simulink model "Linearization"  (R2022a)
settings: Solver=VariableStepAuto  StartTime=0.0  StopTime=100  RelTol=1e-3
undefined symbols (not defined in the file): Aactuator, ac, AeroCoeff, ControlAllocation, DUmax, DUmin, EngineTable, F, fcs, ft, g, hground, IC, kg, LandingGear, Light, LPmethod, m, MIL, Mode_deflection_aileron, Mode_deflection_elevator, Mode_deflection_rudder, Mode_deflection_TVC_y, Mode_deflection_TVC_z, N, Ninv_2nozzle, Ninv_no_nozzle, PIController, s, Sensor, slug, state0, sysID_DAQ, sysID_OBES, Umax_2nozzle, Umax_no_nozzle, Umin_2nozzle, Umin_no_nozzle, WMM2020
libraries: aerolibconvert2 x19, slpidlib x6, simulink x6, sharedutil x4, aerolibatmos2 x3, aerolibwind2 x3, aerolibbdyn x3, aerolibgravity2 x2, sharedtransform x1
(part 1 of 9)
settings Model: Creator=user  LastModifiedBy=user
settings DataIOCC: ExternalInput=getinputstruct(op_trim1)  InitialState=getstatestruct(op_trim1)  LoadExternalInput=on  LoadInitialState=on  ReturnWorkspaceOutputs=off

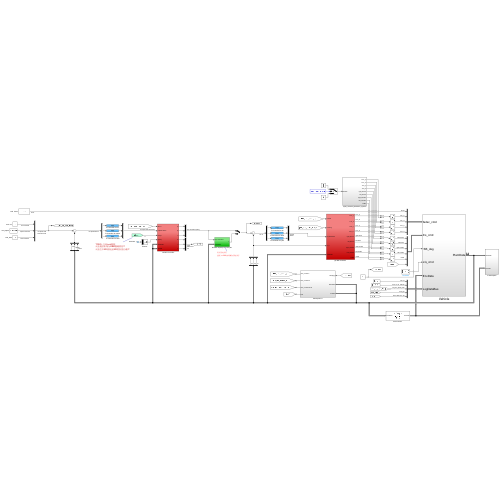
[thumbnail: Simulink's stored preview of the top-level diagram]
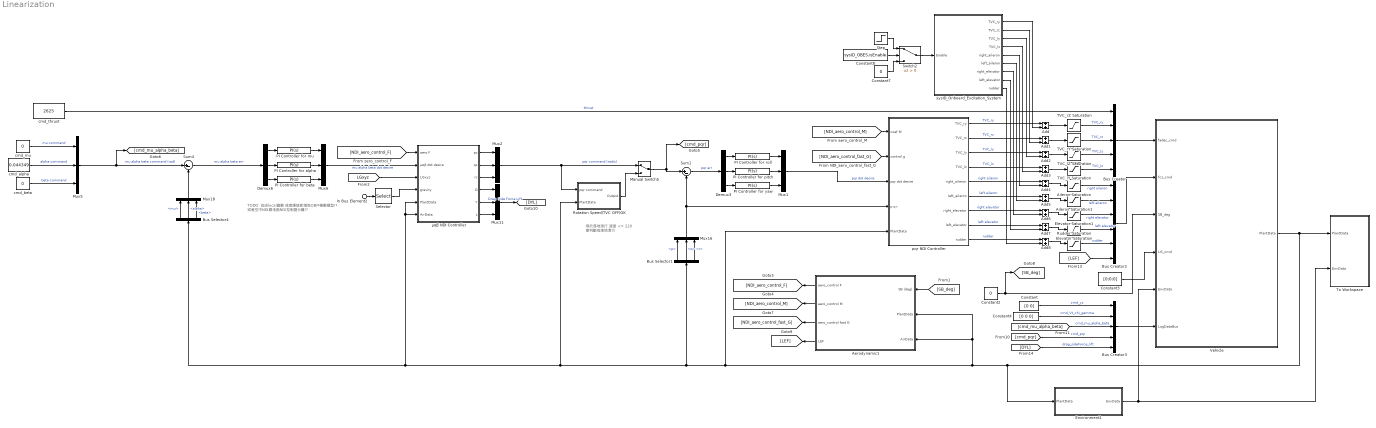
== system Linearization ==
  note: 用於落地滑行
      | 速度 <= 220 會判斷為落地滑行
  note: TODO: 改成local變數
      | 或者應該新增為OBM機載模型!?
      | 或者空中NDI跟地面NDI控制器分離!?
  In Bus Element2 : Inport  PortName=EnvData  Element=g
  Add{,1..8} (9 alike) : Sum
  Aerodynamic1 : Subsystem
  Aileron Saturation : Saturate  UpperLimit=Aactuator.aileron.AngleLimitUpper  LowerLimit=Aactuator.aileron.AngleLimitLower
  Aileron Saturation1 : Saturate  UpperLimit=Aactuator.aileron.AngleLimitUpper  LowerLimit=Aactuator.aileron.AngleLimitLower
  Bus Creator : BusCreator  Inputs=5
  Bus Creator2 : BusCreator  Inputs=6
  Bus Creator3 : BusCreator  Inputs=5
  Bus Selector1 : BusSelector  OutputSignals=p,q,r
  Bus Selector4 : BusSelector  OutputSignals=mu,alpha,beta
  Constant : Constant  Value=[0 0]
  Constant2 : Constant  Value=0
  Constant3 : Constant  Value=[0;0;0]
  Constant4 : Constant  Value=[0 0 0]
  Constant7 : Constant  Value=0
  Constant8 : Constant  Value=sysID_OBES.isEnable
  Demux3 : Demux  Outputs=3
  Demux6 : Demux  Outputs=3
  Elevator Saturation : Saturate  UpperLimit=Aactuator.elevator.AngleLimitUpper  LowerLimit=Aactuator.elevator.AngleLimitLower
  Elevator Saturation1 : Saturate  UpperLimit=Aactuator.elevator.AngleLimitUpper  LowerLimit=Aactuator.elevator.AngleLimitLower
  Environment1 : Subsystem
      mask Display:
      | image('aeroenvironment.bmp','center')
      | % 左側 "Icon transparency" 欄位已選擇 "Opaque with ports"，所以埠名稱會自動顯示，不用再宣告
      | % port_label('input',1,'PlantData')
      | % port_label('output',1,'EnvData')
  Manual Switch5 : ManualSwitch
  Mux{1..2,5..6,11,16,18} (7 alike) : Mux  Inputs=3
  PI Controller for alpha : slpidlib/PID Controller  Controller=PI  Form=Parallel  TimeDomain=Continuous-time  UseExternalTs=off  SampleTime=-1  IntegratorMethod=Forward Euler  FilterMethod=Forward Euler  ControllerParametersSource=internal  P=PIController.alpha.P  I=PIController.alpha.I  UseKiTs=off  D=0  N=100  UseFilter=on  TunerSelectOption=Transfer Function Based (PID Tuner App)  InitialConditionSource=internal  InitialConditionForIntegrator=0  InitialConditionForFilter=0  DifferentiatorICPrevScaledInput=0  ExternalReset=none  TrackingMode=off  Kt=1  LimitOutput=off  SatLimitsSource=internal  UpperSaturationLimit=inf  LowerSaturationLimit=-inf  LinearizeAsGain=on  AntiWindupMode=none  Kb=1  POutMin=[]  POutMax=[]  IOutMin=[]  IOutMax=[]  DOutMin=[]  DOutMax=[]  NOutMin=[]  NOutMax=[]  SumOutMin=[]  SumOutMax=[]  SaturationOutMin=[]  SaturationOutMax=[]  PParamMin=[]  PParamMax=[]  IParamMin=[]  IParamMax=[]  DParamMin=[]  DParamMax=[]  NParamMin=[]  NParamMax=[]  KbParamMin=[]  KbParamMax=[]  KtParamMin=[]  KtParamMax=[]  KbOutMin=[]  KbOutMax=[]  KtOutMin=[]  KtOutMax=[]  IntegratorOutMin=[]  IntegratorOutMax=[]  FilterOutMin=[]  FilterOutMax=[]  SumI1OutMin=[]  SumI1OutMax=[]  SumI2OutMin=[]  SumI2OutMax=[]  SumI3OutMin=[]  SumI3OutMax=[]  SumI4OutMin=[]  SumI4OutMax=[]  SumDOutMin=[]  SumDOutMax=[]  DifferentiatorOutMin=[]  DifferentiatorOutMax=[]  FilterDiffOutCoefMin=[]  FilterDiffOutCoefMax=[]  ReciprocalOutMin=[]  ReciprocalOutMax=[]  SumDenOutMin=[]  SumDenOutMax=[]  SumNumOutMin=[]  SumNumOutMax=[]  DivideOutMin=[]  DivideOutMax=[]  UdiffTsProdOutMin=[]  UdiffTsProdOutMax=[]  NTsProdOutMin=[]  NTsProdOutMax=[]  UintegralTsProdOutMin=[]  UintegralTsProdOutMax=[]  UngainTsProdOutMin=[]  UngainTsProdOutMax=[]  IntegratorContinuousStateAttributes=''  IntegratorStateMustResolveToSignalObject=off  IntegratorRTWStateStorageClass=Auto  FilterContinuousStateAttributes=''  FilterStateMustResolveToSignalObject=off  FilterRTWStateStorageClass=Auto  ParallelPVariant=InternalParameters  IdealPVariant=Disabled  IVariant=InternalParameters  DVariant=Disabled  IntegratorVariant=Continuous  SatVariant=Disabled  AWVariant=Passthrough  PCopyVariant=Disabled  TRVariant=Disabled  FdbkBlocksVariant=Forward  IdealPFdbkVariant=Disabled  SatFdbkVariant=Disabled  DerivativeFilterVariant=Disabled  NVariant=Disabled  NCopyVariant=Disabled_SignalSpec  FilterICVariant=Disabled  IntegratorICVariant=InternalICs  ExternalResetVariant=Disabled  TRSumVariant=Passthrough  SumFdbkVariant=Disabled  SumVariant=Sum_PI  TsampFilterVariant=InternalTs  TsampNgainVariant=Passthrough  TsampIntegralVariant=Passthrough  ExternalSaturationOutDataTypeStr=Inherit: Same as second input  aMode=0
  PI Controller for beta : slpidlib/PID Controller  Controller=PI  Form=Parallel  TimeDomain=Continuous-time  UseExternalTs=off  SampleTime=-1  IntegratorMethod=Forward Euler  FilterMethod=Forward Euler  ControllerParametersSource=internal  P=PIController.beta.P  I=PIController.beta.I  UseKiTs=off  D=0  N=100  UseFilter=on  TunerSelectOption=Transfer Function Based (PID Tuner App)  InitialConditionSource=internal  InitialConditionForIntegrator=0  InitialConditionForFilter=0  DifferentiatorICPrevScaledInput=0  ExternalReset=none  TrackingMode=off  Kt=1  LimitOutput=off  SatLimitsSource=internal  UpperSaturationLimit=inf  LowerSaturationLimit=-inf  LinearizeAsGain=on  AntiWindupMode=none  Kb=1  POutMin=[]  POutMax=[]  IOutMin=[]  IOutMax=[]  DOutMin=[]  DOutMax=[]  NOutMin=[]  NOutMax=[]  SumOutMin=[]  SumOutMax=[]  SaturationOutMin=[]  SaturationOutMax=[]  PParamMin=[]  PParamMax=[]  IParamMin=[]  IParamMax=[]  DParamMin=[]  DParamMax=[]  NParamMin=[]  NParamMax=[]  KbParamMin=[]  KbParamMax=[]  KtParamMin=[]  KtParamMax=[]  KbOutMin=[]  KbOutMax=[]  KtOutMin=[]  KtOutMax=[]  IntegratorOutMin=[]  IntegratorOutMax=[]  FilterOutMin=[]  FilterOutMax=[]  SumI1OutMin=[]  SumI1OutMax=[]  SumI2OutMin=[]  SumI2OutMax=[]  SumI3OutMin=[]  SumI3OutMax=[]  SumI4OutMin=[]  SumI4OutMax=[]  SumDOutMin=[]  SumDOutMax=[]  DifferentiatorOutMin=[]  DifferentiatorOutMax=[]  FilterDiffOutCoefMin=[]  FilterDiffOutCoefMax=[]  ReciprocalOutMin=[]  ReciprocalOutMax=[]  SumDenOutMin=[]  SumDenOutMax=[]  SumNumOutMin=[]  SumNumOutMax=[]  DivideOutMin=[]  DivideOutMax=[]  UdiffTsProdOutMin=[]  UdiffTsProdOutMax=[]  NTsProdOutMin=[]  NTsProdOutMax=[]  UintegralTsProdOutMin=[]  UintegralTsProdOutMax=[]  UngainTsProdOutMin=[]  UngainTsProdOutMax=[]  IntegratorContinuousStateAttributes=''  IntegratorStateMustResolveToSignalObject=off  IntegratorRTWStateStorageClass=Auto  FilterContinuousStateAttributes=''  FilterStateMustResolveToSignalObject=off  FilterRTWStateStorageClass=Auto  ParallelPVariant=InternalParameters  IdealPVariant=Disabled  IVariant=InternalParameters  DVariant=Disabled  IntegratorVariant=Continuous  SatVariant=Disabled  AWVariant=Passthrough  PCopyVariant=Disabled  TRVariant=Disabled  FdbkBlocksVariant=Forward  IdealPFdbkVariant=Disabled  SatFdbkVariant=Disabled  DerivativeFilterVariant=Disabled  NVariant=Disabled  NCopyVariant=Disabled_SignalSpec  FilterICVariant=Disabled  IntegratorICVariant=InternalICs  ExternalResetVariant=Disabled  TRSumVariant=Passthrough  SumFdbkVariant=Disabled  SumVariant=Sum_PI  TsampFilterVariant=InternalTs  TsampNgainVariant=Passthrough  TsampIntegralVariant=Passthrough  ExternalSaturationOutDataTypeStr=Inherit: Same as second input  aMode=0
  PI Controller for mu : slpidlib/PID Controller  Controller=PI  Form=Parallel  TimeDomain=Continuous-time  UseExternalTs=off  SampleTime=-1  IntegratorMethod=Forward Euler  FilterMethod=Forward Euler  ControllerParametersSource=internal  P=PIController.mu.P  I=PIController.mu.I  UseKiTs=off  D=0  N=100  UseFilter=on  TunerSelectOption=Transfer Function Based (PID Tuner App)  InitialConditionSource=internal  InitialConditionForIntegrator=0  InitialConditionForFilter=0  DifferentiatorICPrevScaledInput=0  ExternalReset=none  TrackingMode=off  Kt=1  LimitOutput=off  SatLimitsSource=internal  UpperSaturationLimit=inf  LowerSaturationLimit=-inf  LinearizeAsGain=on  AntiWindupMode=none  Kb=1  POutMin=[]  POutMax=[]  IOutMin=[]  IOutMax=[]  DOutMin=[]  DOutMax=[]  NOutMin=[]  NOutMax=[]  SumOutMin=[]  SumOutMax=[]  SaturationOutMin=[]  SaturationOutMax=[]  PParamMin=[]  PParamMax=[]  IParamMin=[]  IParamMax=[]  DParamMin=[]  DParamMax=[]  NParamMin=[]  NParamMax=[]  KbParamMin=[]  KbParamMax=[]  KtParamMin=[]  KtParamMax=[]  KbOutMin=[]  KbOutMax=[]  KtOutMin=[]  KtOutMax=[]  IntegratorOutMin=[]  IntegratorOutMax=[]  FilterOutMin=[]  FilterOutMax=[]  SumI1OutMin=[]  SumI1OutMax=[]  SumI2OutMin=[]  SumI2OutMax=[]  SumI3OutMin=[]  SumI3OutMax=[]  SumI4OutMin=[]  SumI4OutMax=[]  SumDOutMin=[]  SumDOutMax=[]  DifferentiatorOutMin=[]  DifferentiatorOutMax=[]  FilterDiffOutCoefMin=[]  FilterDiffOutCoefMax=[]  ReciprocalOutMin=[]  ReciprocalOutMax=[]  SumDenOutMin=[]  SumDenOutMax=[]  SumNumOutMin=[]  SumNumOutMax=[]  DivideOutMin=[]  DivideOutMax=[]  UdiffTsProdOutMin=[]  UdiffTsProdOutMax=[]  NTsProdOutMin=[]  NTsProdOutMax=[]  UintegralTsProdOutMin=[]  UintegralTsProdOutMax=[]  UngainTsProdOutMin=[]  UngainTsProdOutMax=[]  IntegratorContinuousStateAttributes=''  IntegratorStateMustResolveToSignalObject=off  IntegratorRTWStateStorageClass=Auto  FilterContinuousStateAttributes=''  FilterStateMustResolveToSignalObject=off  FilterRTWStateStorageClass=Auto  ParallelPVariant=InternalParameters  IdealPVariant=Disabled  IVariant=InternalParameters  DVariant=Disabled  IntegratorVariant=Continuous  SatVariant=Disabled  AWVariant=Passthrough  PCopyVariant=Disabled  TRVariant=Disabled  FdbkBlocksVariant=Forward  IdealPFdbkVariant=Disabled  SatFdbkVariant=Disabled  DerivativeFilterVariant=Disabled  NVariant=Disabled  NCopyVariant=Disabled_SignalSpec  FilterICVariant=Disabled  IntegratorICVariant=InternalICs  ExternalResetVariant=Disabled  TRSumVariant=Passthrough  SumFdbkVariant=Disabled  SumVariant=Sum_PI  TsampFilterVariant=InternalTs  TsampNgainVariant=Passthrough  TsampIntegralVariant=Passthrough  ExternalSaturationOutDataTypeStr=Inherit: Same as second input  aMode=0
  PI Controller for pitch : slpidlib/PID Controller  Controller=PI  Form=Parallel  TimeDomain=Continuous-time  UseExternalTs=off  SampleTime=-1  IntegratorMethod=Forward Euler  FilterMethod=Forward Euler  ControllerParametersSource=internal  P=PIController.q.P  I=PIController.q.I  UseKiTs=off  D=0  N=100  UseFilter=on  TunerSelectOption=Transfer Function Based (PID Tuner App)  InitialConditionSource=internal  InitialConditionForIntegrator=0  InitialConditionForFilter=0  DifferentiatorICPrevScaledInput=0  ExternalReset=none  TrackingMode=off  Kt=1  LimitOutput=off  SatLimitsSource=internal  UpperSaturationLimit=inf  LowerSaturationLimit=-inf  LinearizeAsGain=on  AntiWindupMode=none  Kb=1  POutMin=[]  POutMax=[]  IOutMin=[]  IOutMax=[]  DOutMin=[]  DOutMax=[]  NOutMin=[]  NOutMax=[]  SumOutMin=[]  SumOutMax=[]  SaturationOutMin=[]  SaturationOutMax=[]  PParamMin=[]  PParamMax=[]  IParamMin=[]  IParamMax=[]  DParamMin=[]  DParamMax=[]  NParamMin=[]  NParamMax=[]  KbParamMin=[]  KbParamMax=[]  KtParamMin=[]  KtParamMax=[]  KbOutMin=[]  KbOutMax=[]  KtOutMin=[]  KtOutMax=[]  IntegratorOutMin=[]  IntegratorOutMax=[]  FilterOutMin=[]  FilterOutMax=[]  SumI1OutMin=[]  SumI1OutMax=[]  SumI2OutMin=[]  SumI2OutMax=[]  SumI3OutMin=[]  SumI3OutMax=[]  SumI4OutMin=[]  SumI4OutMax=[]  SumDOutMin=[]  SumDOutMax=[]  DifferentiatorOutMin=[]  DifferentiatorOutMax=[]  FilterDiffOutCoefMin=[]  FilterDiffOutCoefMax=[]  ReciprocalOutMin=[]  ReciprocalOutMax=[]  SumDenOutMin=[]  SumDenOutMax=[]  SumNumOutMin=[]  SumNumOutMax=[]  DivideOutMin=[]  DivideOutMax=[]  UdiffTsProdOutMin=[]  UdiffTsProdOutMax=[]  NTsProdOutMin=[]  NTsProdOutMax=[]  UintegralTsProdOutMin=[]  UintegralTsProdOutMax=[]  UngainTsProdOutMin=[]  UngainTsProdOutMax=[]  IntegratorContinuousStateAttributes=''  IntegratorStateMustResolveToSignalObject=off  IntegratorRTWStateStorageClass=Auto  FilterContinuousStateAttributes=''  FilterStateMustResolveToSignalObject=off  FilterRTWStateStorageClass=Auto  ParallelPVariant=InternalParameters  IdealPVariant=Disabled  IVariant=InternalParameters  DVariant=Disabled  IntegratorVariant=Continuous  SatVariant=Disabled  AWVariant=Passthrough  PCopyVariant=Disabled  TRVariant=Disabled  FdbkBlocksVariant=Forward  IdealPFdbkVariant=Disabled  SatFdbkVariant=Disabled  DerivativeFilterVariant=Disabled  NVariant=Disabled  NCopyVariant=Disabled_SignalSpec  FilterICVariant=Disabled  IntegratorICVariant=InternalICs  ExternalResetVariant=Disabled  TRSumVariant=Passthrough  SumFdbkVariant=Disabled  SumVariant=Sum_PI  TsampFilterVariant=InternalTs  TsampNgainVariant=Passthrough  TsampIntegralVariant=Passthrough  ExternalSaturationOutDataTypeStr=Inherit: Same as second input  aMode=0
  PI Controller for roll : slpidlib/PID Controller  Controller=PI  Form=Parallel  TimeDomain=Continuous-time  UseExternalTs=off  SampleTime=-1  IntegratorMethod=Forward Euler  FilterMethod=Forward Euler  ControllerParametersSource=internal  P=PIController.p.P  I=PIController.p.I  UseKiTs=off  D=0  N=100  UseFilter=on  TunerSelectOption=Transfer Function Based (PID Tuner App)  InitialConditionSource=internal  InitialConditionForIntegrator=0  InitialConditionForFilter=0  DifferentiatorICPrevScaledInput=0  ExternalReset=none  TrackingMode=off  Kt=1  LimitOutput=off  SatLimitsSource=internal  UpperSaturationLimit=inf  LowerSaturationLimit=-inf  LinearizeAsGain=on  AntiWindupMode=none  Kb=1  POutMin=[]  POutMax=[]  IOutMin=[]  IOutMax=[]  DOutMin=[]  DOutMax=[]  NOutMin=[]  NOutMax=[]  SumOutMin=[]  SumOutMax=[]  SaturationOutMin=[]  SaturationOutMax=[]  PParamMin=[]  PParamMax=[]  IParamMin=[]  IParamMax=[]  DParamMin=[]  DParamMax=[]  NParamMin=[]  NParamMax=[]  KbParamMin=[]  KbParamMax=[]  KtParamMin=[]  KtParamMax=[]  KbOutMin=[]  KbOutMax=[]  KtOutMin=[]  KtOutMax=[]  IntegratorOutMin=[]  IntegratorOutMax=[]  FilterOutMin=[]  FilterOutMax=[]  SumI1OutMin=[]  SumI1OutMax=[]  SumI2OutMin=[]  SumI2OutMax=[]  SumI3OutMin=[]  SumI3OutMax=[]  SumI4OutMin=[]  SumI4OutMax=[]  SumDOutMin=[]  SumDOutMax=[]  DifferentiatorOutMin=[]  DifferentiatorOutMax=[]  FilterDiffOutCoefMin=[]  FilterDiffOutCoefMax=[]  ReciprocalOutMin=[]  ReciprocalOutMax=[]  SumDenOutMin=[]  SumDenOutMax=[]  SumNumOutMin=[]  SumNumOutMax=[]  DivideOutMin=[]  DivideOutMax=[]  UdiffTsProdOutMin=[]  UdiffTsProdOutMax=[]  NTsProdOutMin=[]  NTsProdOutMax=[]  UintegralTsProdOutMin=[]  UintegralTsProdOutMax=[]  UngainTsProdOutMin=[]  UngainTsProdOutMax=[]  IntegratorContinuousStateAttributes=''  IntegratorStateMustResolveToSignalObject=off  IntegratorRTWStateStorageClass=Auto  FilterContinuousStateAttributes=''  FilterStateMustResolveToSignalObject=off  FilterRTWStateStorageClass=Auto  ParallelPVariant=InternalParameters  IdealPVariant=Disabled  IVariant=InternalParameters  DVariant=Disabled  IntegratorVariant=Continuous  SatVariant=Disabled  AWVariant=Passthrough  PCopyVariant=Disabled  TRVariant=Disabled  FdbkBlocksVariant=Forward  IdealPFdbkVariant=Disabled  SatFdbkVariant=Disabled  DerivativeFilterVariant=Disabled  NVariant=Disabled  NCopyVariant=Disabled_SignalSpec  FilterICVariant=Disabled  IntegratorICVariant=InternalICs  ExternalResetVariant=Disabled  TRSumVariant=Passthrough  SumFdbkVariant=Disabled  SumVariant=Sum_PI  TsampFilterVariant=InternalTs  TsampNgainVariant=Passthrough  TsampIntegralVariant=Passthrough  ExternalSaturationOutDataTypeStr=Inherit: Same as second input  aMode=0
  PI Controller for yaw : slpidlib/PID Controller  Controller=PI  Form=Parallel  TimeDomain=Continuous-time  UseExternalTs=off  SampleTime=-1  IntegratorMethod=Forward Euler  FilterMethod=Forward Euler  ControllerParametersSource=internal  P=PIController.r.P  I=PIController.r.I  UseKiTs=off  D=0  N=100  UseFilter=on  TunerSelectOption=Transfer Function Based (PID Tuner App)  InitialConditionSource=internal  InitialConditionForIntegrator=0  InitialConditionForFilter=0  DifferentiatorICPrevScaledInput=0  ExternalReset=none  TrackingMode=off  Kt=1  LimitOutput=off  SatLimitsSource=internal  UpperSaturationLimit=inf  LowerSaturationLimit=-inf  LinearizeAsGain=on  AntiWindupMode=none  Kb=1  POutMin=[]  POutMax=[]  IOutMin=[]  IOutMax=[]  DOutMin=[]  DOutMax=[]  NOutMin=[]  NOutMax=[]  SumOutMin=[]  SumOutMax=[]  SaturationOutMin=[]  SaturationOutMax=[]  PParamMin=[]  PParamMax=[]  IParamMin=[]  IParamMax=[]  DParamMin=[]  DParamMax=[]  NParamMin=[]  NParamMax=[]  KbParamMin=[]  KbParamMax=[]  KtParamMin=[]  KtParamMax=[]  KbOutMin=[]  KbOutMax=[]  KtOutMin=[]  KtOutMax=[]  IntegratorOutMin=[]  IntegratorOutMax=[]  FilterOutMin=[]  FilterOutMax=[]  SumI1OutMin=[]  SumI1OutMax=[]  SumI2OutMin=[]  SumI2OutMax=[]  SumI3OutMin=[]  SumI3OutMax=[]  SumI4OutMin=[]  SumI4OutMax=[]  SumDOutMin=[]  SumDOutMax=[]  DifferentiatorOutMin=[]  DifferentiatorOutMax=[]  FilterDiffOutCoefMin=[]  FilterDiffOutCoefMax=[]  ReciprocalOutMin=[]  ReciprocalOutMax=[]  SumDenOutMin=[]  SumDenOutMax=[]  SumNumOutMin=[]  SumNumOutMax=[]  DivideOutMin=[]  DivideOutMax=[]  UdiffTsProdOutMin=[]  UdiffTsProdOutMax=[]  NTsProdOutMin=[]  NTsProdOutMax=[]  UintegralTsProdOutMin=[]  UintegralTsProdOutMax=[]  UngainTsProdOutMin=[]  UngainTsProdOutMax=[]  IntegratorContinuousStateAttributes=''  IntegratorStateMustResolveToSignalObject=off  IntegratorRTWStateStorageClass=Auto  FilterContinuousStateAttributes=''  FilterStateMustResolveToSignalObject=off  FilterRTWStateStorageClass=Auto  ParallelPVariant=InternalParameters  IdealPVariant=Disabled  IVariant=InternalParameters  DVariant=Disabled  IntegratorVariant=Continuous  SatVariant=Disabled  AWVariant=Passthrough  PCopyVariant=Disabled  TRVariant=Disabled  FdbkBlocksVariant=Forward  IdealPFdbkVariant=Disabled  SatFdbkVariant=Disabled  DerivativeFilterVariant=Disabled  NVariant=Disabled  NCopyVariant=Disabled_SignalSpec  FilterICVariant=Disabled  IntegratorICVariant=InternalICs  ExternalResetVariant=Disabled  TRSumVariant=Passthrough  SumFdbkVariant=Disabled  SumVariant=Sum_PI  TsampFilterVariant=InternalTs  TsampNgainVariant=Passthrough  TsampIntegralVariant=Passthrough  ExternalSaturationOutDataTypeStr=Inherit: Same as second input  aMode=0
  Rotation Speed(TVC OFF)OK : Subsystem
  Rudder Saturation : Saturate  UpperLimit=Aactuator.rudder.AngleLimitUpper  LowerLimit=Aactuator.rudder.AngleLimitLower
  Selector : Selector  InputPortWidth=3  IndexOptions=Index vector (dialog)  Indices=3  OutputSizes=1
  Step : Step  Time=sysID_OBES.start_time  SampleTime=0
  Sum1 : Sum  Inputs=|+-
  Sum4 : Sum  Inputs=|+-
  Switch2 : Switch  Criteria=u2 > Threshold  SaturateOnIntegerOverflow=off  InputSameDT=off
  TVC_lY Saturation : Saturate  UpperLimit=Aactuator.TVC_Z.AngleLimitUpper  LowerLimit=Aactuator.TVC_Z.AngleLimitLower
  TVC_lZ Saturation : Saturate  UpperLimit=Aactuator.TVC_Y.AngleLimitUpper  LowerLimit=Aactuator.TVC_Y.AngleLimitLower
  TVC_rY Saturation : Saturate  UpperLimit=Aactuator.TVC_Z.AngleLimitUpper  LowerLimit=Aactuator.TVC_Z.AngleLimitLower
  TVC_rZ Saturation : Saturate  UpperLimit=Aactuator.TVC_Y.AngleLimitUpper  LowerLimit=Aactuator.TVC_Y.AngleLimitLower
  To Workspace : Subsystem
  Vehicle : Subsystem
  cmd_alpha : Constant  Value=0.044349
  cmd_beta : Constant  Value=0
  cmd_mu : Constant  Value=0
  cmd_thrust : Constant  Value=2625
  pqr NDI Controller : Subsystem  VariantControl=TVC ON
  sysID_Onboard_Excitation_System : Subsystem
  μαβ NDI Controller : Subsystem
  wires:
  Rudder Saturation/1 -> Bus Creator2/5  "rudder"
  Vehicle/1(PlantData) -> Environment1/1(PlantData), μαβ NDI Controller/5(PlantData), μαβ NDI Controller/6(AirData), Bus Selector4/1, Rotation Speed(TVC OFF)OK/2(PlantData), Bus Selector1/1, pqr NDI Controller/5(PlantData), Aerodynamic1/2(PlantData), Aerodynamic1/3(AirData), To Workspace/1(PlantData)
  Add3/1 -> TVC_lY Saturation/1
  Constant8/1 -> Switch2/2
  μαβ NDI Controller/5(Y) -> Mux11/2
  [LEF] -> Bus Creator2/6
  Manual Switch5/1 -> [cmd_pqr], Sum1/1
  Mux1/1 -> pqr NDI Controller/3(pqr dot desire)  "pqr dot desire"
  Add1/1 -> TVC_rY Saturation/1
  pqr NDI Controller/3("TVC_ly ") -> Add2/1  "TVC_ly"
  Rotation Speed(TVC OFF)OK/1(Output) -> Manual Switch5/2
  μαβ NDI Controller/6(L) -> Mux11/3
  [NDI_aero_control_fast_G] -> pqr NDI Controller/2(control g)
  pqr NDI Controller/8(left_elevator) -> Add7/1  "left elevator"
  pqr NDI Controller/5(right_aileron) -> Add4/1  "right aileron"
  [NDI_aero_control_F] -> μαβ NDI Controller/1(aero F)
  [NDI_aero_control_M] -> pqr NDI Controller/1(coef M)
  pqr NDI Controller/2(TVC_rz) -> Add1/1  "TVC_rz"
  Bus Selector1/1 -> Mux16/1  "<p>"
  Step/1 -> Switch2/1
  Mux2/1 -> Manual Switch5/1, Rotation Speed(TVC OFF)OK/1(pqr command)  "pqr command (rad/s)"
  TVC_lY Saturation/1 -> Bus Creator/5  "TVC_lz"
  Add7/1 -> Elevator Saturation/1
  Add2/1 -> TVC_lZ Saturation/1
  Demux6/2 -> PI Controller for alpha/1
  pqr NDI Controller/7(right_elevator) -> Add6/1  "right elevator"
  pqr NDI Controller/6(left_aileron) -> Add5/1  "left aileron"
  Add5/1 -> Aileron Saturation1/1
  μαβ NDI Controller/3(rc) -> Mux2/3
  pqr NDI Controller/1("TVC_ry ") -> Add/1  "TVC_ry"
  Add/1 -> TVC_rZ Saturation/1
  sysID_Onboard_Excitation_System/4(TVC_lz) -> Add3/2
  TVC_rY Saturation/1 -> Bus Creator/3  "TVC_rz"
  sysID_Onboard_Excitation_System/2(TVC_rz) -> Add1/2
  Constant7/1 -> Switch2/3
  Switch2/1 -> sysID_Onboard_Excitation_System/1(Enable)
  Add4/1 -> Aileron Saturation/1
  sysID_Onboard_Excitation_System/9(rudder) -> Add8/2
  Aileron Saturation1/1 -> Bus Creator2/2  "left aileron"
  [LGxyz] -> μαβ NDI Controller/3(LGxyz)
  PI Controller for mu/1 -> Mux6/1
  TVC_lZ Saturation/1 -> Bus Creator/4  "TVC_ly"
  Elevator Saturation1/1 -> Bus Creator2/3  "right elevator"
  Bus Creator2/1 -> Vehicle/2(fcs_cmd)
  TVC_rZ Saturation/1 -> Bus Creator/2  "TVC_ry"
  Elevator Saturation/1 -> Bus Creator2/4  "left elevator"
  Bus Creator/1 -> Vehicle/1(fadec_cmd)
  sysID_Onboard_Excitation_System/8(left_elevator) -> Add7/2
  μαβ NDI Controller/4(D) -> Mux11/1
  μαβ NDI Controller/2(qc) -> Mux2/2
  sysID_Onboard_Excitation_System/1(TVC_ry) -> Add/2
  Add8/1 -> Rudder Saturation/1
  Bus Selector4/1 -> Mux18/1  "<mu>"
  Aerodynamic1/4(LEF) -> [LEF]
  PI Controller for alpha/1 -> Mux6/2
  Demux3/3 -> PI Controller for yaw/1
  sysID_Onboard_Excitation_System/7(right_elevator) -> Add6/2
  Demux6/1 -> PI Controller for mu/1
  Mux6/1 -> μαβ NDI Controller/2(μαβ dot desire)  "mu alpha beta dot desire"
  Bus Selector1/2 -> Mux16/2  "<q>"
  Bus Selector4/2 -> Mux18/2  "<alpha>"
  Add6/1 -> Elevator Saturation1/1
  Aerodynamic1/2(aero_control M) -> [NDI_aero_control_M]
  Mux18/1 -> Sum4/2
  Mux11/1 -> [DYL]  "Drag  Side Force Lift"
  Demux6/3 -> PI Controller for beta/1
  sysID_Onboard_Excitation_System/3(TVC_ly) -> Add2/2
  Demux3/1 -> PI Controller for roll/1
  [SB_deg] -> Aerodynamic1/1(SB (deg))
  Sum1/1 -> Demux3/1  "pqr err"
  PI Controller for beta/1 -> Mux6/3
  Mux16/1 -> pqr NDI Controller/4(p q r), Sum1/2
  sysID_Onboard_Excitation_System/5(right_aileron) -> Add4/2
  In Bus Element2/1 -> Selector/1
  Selector/1 -> μαβ NDI Controller/4(gravity)
  Bus Selector1/3 -> Mux16/3  "<r>"
  Bus Selector4/3 -> Mux18/3  "<beta>"
  Sum4/1 -> Demux6/1  "mu alpha beta err"
  pqr NDI Controller/4("TVC_lz ") -> Add3/1  "TVC_lz"
  Mux5/1 -> [cmd_mu_alpha_beta], Sum4/1  "mu alpha beta command (rad)"
  sysID_Onboard_Excitation_System/6(left_aileron) -> Add5/2
  PI Controller for pitch/1 -> Mux1/2
  PI Controller for yaw/1 -> Mux1/3
  Aerodynamic1/1(aero_control F) -> [NDI_aero_control_F]
  Aileron Saturation/1 -> Bus Creator2/1  "right aileron"
  PI Controller for roll/1 -> Mux1/1
  μαβ NDI Controller/1(pc) -> Mux2/1
  Demux3/2 -> PI Controller for pitch/1
  Aerodynamic1/3(aero_control fast G) -> [NDI_aero_control_fast_G]
  pqr NDI Controller/9(rudder) -> Add8/1  "rudder"
  Constant2/1 -> [SB_deg], Vehicle/3(" SB_deg")
  [cmd_mu_alpha_beta] -> Bus Creator3/3  "cmd_mu_alpha_beta"
  Bus Creator3/1 -> Vehicle/6(LogDataBus)
  Constant/1 -> Bus Creator3/1  "cmd_yz"
  Constant4/1 -> Bus Creator3/2  "cmd_Vt_chi_gamma"
  [cmd_pqr] -> Bus Creator3/4  "cmd_pqr"
  [DYL] -> Bus Creator3/5  "drag_sideForce_lift"
  Constant3/1 -> Vehicle/4(LG_cmd)
  cmd_beta/1 -> Mux5/3  "beta command"
  cmd_alpha/1 -> Mux5/2  "alpha command"
  cmd_mu/1 -> Mux5/1  "mu command"
  cmd_thrust/1 -> Bus Creator/1  "thrust"
  Environment1/1(EnvData) -> To Workspace/2(EnvData), Vehicle/5(EnvData)

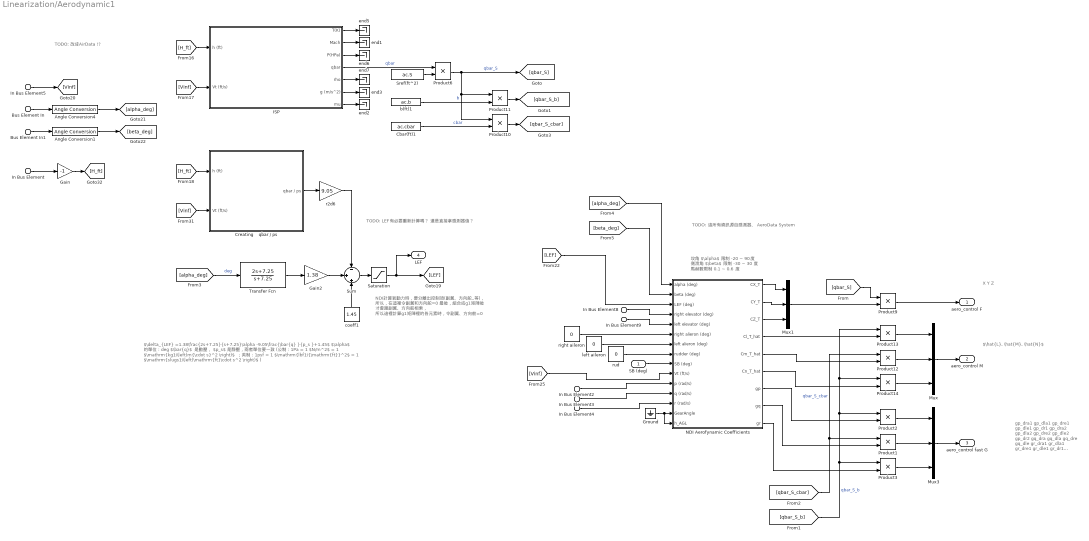
== system Linearization/Aerodynamic1 ==
  note: NDI計算氣動力時，要分離出控制項(副翼、方向舵..等)，
      | 所以，在這裡令副翼和方向舵=0
      | 最後，組合成g1矩陣後 才會跟副翼、方向舵相乘，
      | 所以這裡計算g1矩陣裡的各元素時，令副翼、方向舵=0
  note: TODO: LEF有必要重新計算嗎？
      | 還是直接拿感測器值？
  note: X
      | Y
      | Z
  note: $\delta_{LEF} =1.38\frac{2s+7.25}{s+7.25}\alpha -9.05\frac{\bar{q} }{p_s }+1.45$
      | $\alpha$ 的單位：deg
      | $\bar{q}$ 是動壓， $p_s$ 是靜壓，兩者單位要一致 (公制：1Pa = 1 $N/m^2$ = 1 $\mathrm{kg}/\left(m{\cdot s}^2 \right)$ ；英制：1psf = 1 $\mathrm{lbf}/{\mathrm{ft}}^2$ = 1 $\mathrm{slugs}/\left(\mathrm{ft}\cdot s^2 \right)$ )
  note: $\hat{L}, \hat{M}, \hat{N}$
  note: TODO: 這所有資訊源自感測器、
      | AeroData System
  note: TODO: 改成AirData !?
  note: 攻角 $\alpha$ 限制 -20 ~ 90度
      | 側滑角 $\beta$ 限制 -30 ~ 30 度
      | 馬赫數限制 0.1 ~ 0.6 度
  note: gp_dra1
      | gp_dla1
      | gp_dre1
      | gp_dle1
      | gp_dr1
      | gp_dra2
      | gp_dla2
      | gp_dre2
      | gp_dle2
      | gp_dr2
      |
      | gq_dra
      | gq_dla
      | gq_dre
      | gq_dle
      |
      | gr_dra1
      | gr_dla1
      | gr_dre1
      | gr_dle1
      | gr_dr1
      | gr_dra2
      | gr_dla2
      | gr_dre2
      | gr_dle2
      | gr_dr2
  SB (deg) : Inport  Unit=deg
  In Bus Element : Inport  Port=2  PortName=PlantData  Element=altitude
  In Bus Element8 : Inport  Port=2  PortName=PlantData  Element=AeroActBus.right Elevator_deg
  In Bus Element9 : Inport  Port=2  PortName=PlantData  Element=AeroActBus.left Elevator_deg
  In Bus Element2 : Inport  Port=2  PortName=PlantData  Element=p
  In Bus Element3 : Inport  Port=2  PortName=PlantData  Element=q
  In Bus Element4 : Inport  Port=2  PortName=PlantData  Element=r
  In Bus Element5 : Inport  Port=2  PortName=PlantData  Element=Vt
  Bus Element In : Inport  Port=3  PortName=AirData  Element=alpha
  Bus Element In1 : Inport  Port=3  PortName=AirData  Element=beta
  Angle Conversion1 : aerolibconvert2/Angle Conversion  IU=rad  OU=deg
  Angle Conversion4 : aerolibconvert2/Angle Conversion  IU=rad  OU=deg
  Cbar(ft)1 : Constant  Value=ac.cbar
  Creating    qbar / ps : Subsystem
  Gain : Gain  Gain=-1
  Gain2 : Gain  Gain=1.38  SaturateOnIntegerOverflow=on  OutDataTypeStr=Inherit: Same as input  ParamDataTypeStr=Inherit: Same as input
  Ground : Ground
  "ISP " : Subsystem
  Mux : Mux  Inputs=3
  Mux1 : Mux  Inputs=3
  Mux3 : Mux  Inputs=3
  NDI Aerofynamic Coefficients : Subsystem
  Product{1..3,6,9..14} (10 alike) : Product
  Saturation : Saturate  UpperLimit=Aactuator.LEF.AngleLimitUpper  LowerLimit=Aactuator.LEF.AngleLimitLower
  Sref(ft^2) : Constant  Value=ac.S
  Sum : Sum  Inputs=-|+|+  InputSameDT=on  SaturateOnIntegerOverflow=on  OutDataTypeStr=Inherit: Same as first input
  Transfer Fcn : TransferFcn  Numerator=[2 7.25]  Denominator=[1 7.25]
  b(ft)1 : Constant  Value=ac.b
  coeff1 : Constant  Value=1.45
  end{1..3,5..7} (6 alike) : Terminator
  left aileron : Constant  Value=0
  r2d6 : Gain  Gain=9.05  SaturateOnIntegerOverflow=on  OutDataTypeStr=Inherit: Same as input  ParamDataTypeStr=Inherit: Same as input
  right aileron : Constant  Value=0
  rud : Constant  Value=0
  aero_control F : Outport  VectorParamsAs1DForOutWhenUnconnected=off
  aero_control M : Outport  Port=2  VectorParamsAs1DForOutWhenUnconnected=off
  aero_control fast G : Outport  Port=3  VectorParamsAs1DForOutWhenUnconnected=off
  LEF : Outport  Port=4
  wires:
  [Vinf] -> "ISP "/2(Vt (ft/s))
  "ISP "/2("Mach ") -> end1/1
  "ISP "/7(mu) -> end2/1
  "ISP "/6(g (m/s^2)) -> end3/1
  "ISP "/5(rho) -> end7/1
  "ISP "/4("qbar ") -> Product6/1  "qbar"
  "ISP "/3(P(HPa)) -> end6/1
  "ISP "/1(T(K)) -> end5/1
  r2d6/1 -> Sum/1
  Creating    qbar / ps/1(qbar / ps) -> r2d6/1
  [alpha_deg] -> Transfer Fcn/1  "deg"
  [Vinf] -> Creating    qbar / ps/2(Vt (ft/s))
  coeff1/1 -> Sum/3
  [H_ft] -> Creating    qbar / ps/1(h (ft))
  [H_ft] -> "ISP "/1(h (ft))
  Sum/1 -> Saturation/1
  Saturation/1 -> LEF/1, [LEF]
  Transfer Fcn/1 -> Gain2/1
  In Bus Element/1 -> Gain/1
  Gain/1 -> [H_ft]
  Cbar(ft)1/1 -> Product10/2  "cbar"
  b(ft)1/1 -> Product11/2  "b"
  Sref(ft^2)/1 -> Product6/2
  Product10/1 -> [qbar_S_cbar]
  Product6/1 -> Product11/1, Product10/1, [qbar_S]  "qbar_S"
  Product11/1 -> [qbar_S_b]
  [qbar_S] -> Product9/1
  Product9/1 -> aero_control F/1
  Product12/1 -> Mux/2
  Product13/1 -> Mux/1
  Product14/1 -> Mux/3
  Mux/1 -> aero_control M/1
  NDI Aerofynamic Coefficients/4(Cl_T_hat) -> Product13/2
  NDI Aerofynamic Coefficients/5(Cm_T_hat) -> Product12/2
  NDI Aerofynamic Coefficients/6(Cn_T_hat) -> Product14/2
  NDI Aerofynamic Coefficients/1(CX_T) -> Mux1/1
  NDI Aerofynamic Coefficients/2(CY_T) -> Mux1/2
  NDI Aerofynamic Coefficients/3(CZ_T) -> Mux1/3
  Mux1/1 -> Product9/2
  [qbar_S_b] -> Product13/1, Product14/1, Product2/1, Product3/1  "qbar_S_b"
  Product3/1 -> Mux3/3
  Product1/1 -> Mux3/2
  Product2/1 -> Mux3/1
  NDI Aerofynamic Coefficients/7(gp) -> Product2/2
  [qbar_S_cbar] -> Product12/1, Product1/1  "qbar_S_cbar"
  NDI Aerofynamic Coefficients/9(gr) -> Product3/2
  NDI Aerofynamic Coefficients/8(gq) -> Product1/2
  Mux3/1 -> aero_control fast G/1
  [Vinf] -> NDI Aerofynamic Coefficients/10(Vt (ft/s))
  SB (deg)/1 -> NDI Aerofynamic Coefficients/9(SB (deg))
  [LEF] -> NDI Aerofynamic Coefficients/3(LEF (deg))
  [beta_deg] -> NDI Aerofynamic Coefficients/2(beta (deg))
  [alpha_deg] -> NDI Aerofynamic Coefficients/1(alpha (deg))
  In Bus Element2/1 -> NDI Aerofynamic Coefficients/11(p (rad/s))
  In Bus Element3/1 -> NDI Aerofynamic Coefficients/12(q (rad/s))
  In Bus Element4/1 -> NDI Aerofynamic Coefficients/13(r (rad/s))
  Ground/1 -> NDI Aerofynamic Coefficients/14(GearAngle), NDI Aerofynamic Coefficients/15(h_AGL)
  Gain2/1 -> Sum/2
  Bus Element In/1 -> Angle Conversion4/1
  Angle Conversion4/1 -> [alpha_deg]
  Angle Conversion1/1 -> [beta_deg]
  Bus Element In1/1 -> Angle Conversion1/1
  In Bus Element5/1 -> [Vinf]
  In Bus Element8/1 -> NDI Aerofynamic Coefficients/4(right elevator (deg))
  In Bus Element9/1 -> NDI Aerofynamic Coefficients/5(left elevator (deg))
  right aileron/1 -> NDI Aerofynamic Coefficients/6(right alieron (deg))
  left aileron/1 -> NDI Aerofynamic Coefficients/7(left alieron (deg))
  rud/1 -> NDI Aerofynamic Coefficients/8(rudder (deg))

== system Linearization/Environment1 ==
  note: p, q, r
  note: u, v, w
  note: Wind Models
  note: Atmosphere Model
  note: Altitude must be less than 20000 m (approximately 65620 feet).
  note: 建模注意： EnvData Bus 內要指定公制/英制單位
  note: Magnetic Field
  note: Gravity Model
  note: TODO: 改用這個現成模塊...
      | 但NDI控制器內的重力g是用常數，將產生誤差...
  note: TODO: 改用這個現成模塊...
      | 參考MATLAB Help範例 Quadcopter Project
  note: TODO: 改用現成模塊，改成英制。
      | NDI控制器，不會產生誤差，因為可轉成C程式碼
  note: TODO: 參考MATLAB Help範例 HL-20
      | 將風速效應加到氣動力攻角、側滑角、qbar、Mach、V
  In Bus Element3 : Inport  PortName=PlantData  Element=Vt
  In Bus Element4 : Inport  PortName=PlantData  Element=Vt
  In Bus Element5 : Inport  PortName=PlantData  Element=Vt
  In Bus Element : Inport  PortName=PlantData  Element=DCM_be
  In Bus Element1 : Inport  PortName=PlantData  Element=altitude
  In Bus Element2 : Inport  PortName=PlantData  Element=altitude
  COESA Atmosphere Model : aerolibatmos2/COESA Atmosphere Model  Commented=on  units=English (Velocity in ft/s)  spec=1976 COESA-extended U.S. Standard Atmosphere  model=Profile  profile_var=High temperature  profile_percent=1%  profile_alt=5 km (16404 ft)  envelope_var=High temperature  envelope_percent=1%  action=Warning
  Density Conversion : aerolibconvert2/Density Conversion  IU=kg/m^3  OU=slug/ft^3
      settings: SourceProductBaseCode=AE
  Discrete Wind Gust Model : aerolibwind2/Discrete Wind Gust Model  Commented=on  units=English (Velocity in ft/s)  Gx=on  Gy=on  Gz=on  t_0=5  d_m=[120 120 80]  v_m=[3.5 3.5 3.0]
  Dryden Wind Turbulence Model (Continuous (+q +r)) : aerolibwind2/Dryden Wind Turbulence Model  (Continuous (+q -r))  Commented=on  units=English (Velocity in ft/s)  spec=MIL-F-8785C  model=Continuous Dryden (+q +r)  W20=15  Wdeg=0  TurbProb=10^-2 - Light  L_high=533.4  Wingspan=10  ts=0.1  Seed=[23341 23342 23343 23344]  T_on=on
  Dynamic Pressure : Subsystem
  Geoid Height : aerolibgravity2/Geoid Height  Commented=on  units=English  gtype=EGM96  datafile='geoidegm96grid'  dtype=double  action=Warning
      settings: AttributesFormatString=EGM2008 Geoid Data Unavailable  SourceProductBaseCode=AE
  ISA Atmosphere Model : aerolibatmos2/ISA Atmosphere Model  Commented=on  custom=off  g=9.80665  gamma=1.4  R=287.0531  L=0.0065  h_trop=11000  h_strat=20000  rho0=1.225  P0=101325  T0=288.15  h0=0
  "ISP " : Subsystem
  Length Conversion : aerolibconvert2/Length Conversion  IU=ft  OU=m
  Mach Number : Subsystem
  Magnetic Field : Constant  Value=[0 0 0]
  Manual Switch : ManualSwitch
  Manual Switch1 : ManualSwitch  CurrentSetting=0
  Pressure Altitude : aerolibatmos2/Pressure Altitude  Commented=on  units=English  action=Warning
      settings: SourceProductBaseCode=AE
  Sum : Sum  Commented=on  Inputs=+++
  Velocity Conversion : aerolibconvert2/Velocity Conversion  IU=m/s  OU=ft/s
  "WGS84 Gravity Model  " : GravityWGS84  Commented=on  units=English
  Wind Shear Model : aerolibwind2/Wind Shear Model  Commented=on  units=English (Velocity in ft/s)  phase=Category C - Terminal Flight Phase  W_20=15  Wdeg=0
  World Magnetic Model : aerolibgravity2/World Magnetic Model  Commented=on  model=WMM2020 (2020-2025)  customFile='WMM2020.COF'  units=English  time_in=on  month=January  day=1  year=2020  action=Error  h_out=off  dec_out=off  inc_out=off  ti_out=off
      settings: SourceProductBaseCode=AE
  gravity (ft/s^2) : Constant  Value=g
  hground (ft) : Constant  Value=hground
  no wind : Constant  Value=[0 0 0]
  no wind1 : Constant  Value=[0 0 0]
  r2d1 : Gain  Commented=on  Gain=-1  SaturateOnIntegerOverflow=on  OutDataTypeStr=Inherit: Same as input  ParamDataTypeStr=Inherit: Same as input
  r2d2 : Gain  Gain=-1  SaturateOnIntegerOverflow=on  OutDataTypeStr=Inherit: Same as input  ParamDataTypeStr=Inherit: Same as input
  Out Bus Element : Outport  PortName=EnvData  Element=Pressure
  Out Bus Element1 : Outport  PortName=EnvData  Element=AirDensity
  Out Bus Element2 : Outport  PortName=EnvData  Element=qbar
  Out Bus Element3 : Outport  PortName=EnvData  Element=Mach
  Out Bus Element4 : Outport  PortName=EnvData  Element=g
  Out Bus Element5 : Outport  PortName=EnvData  Element=hground
  Out Bus Element6 : Outport  PortName=EnvData  Element=MagneticField_NED
  Out Bus Element7 : Outport  PortName=EnvData  Element=AirTemperature_K
  Out Bus Element8 : Outport  PortName=EnvData  Element=SoundSpeed_ms
  Out Bus Element9 : Outport  PortName=EnvData  Element=WindVelocity
  Out Bus Element10 : Outport  PortName=EnvData  Element=WindAngularRates
  wires:
  "ISP "/1(T (K)) -> Out Bus Element7/1
  "ISP "/3(P (HPa)) -> Out Bus Element/1
  "ISP "/4(rho (kg/m^3)) -> Density Conversion/1, Out Bus Element1/1
  hground (ft)/1 -> Out Bus Element5/1
  gravity (ft/s^2)/1 -> Out Bus Element4/1  "Gravity_NED"
  Magnetic Field/1 -> Out Bus Element6/1  "MagneticField_NED"
  In Bus Element1/1 -> r2d2/1
  r2d2/1 -> Length Conversion/1  "h(ft)"
  Length Conversion/1 -> "ISP "/1(h(m))
  "ISP "/2(a (m/s)) -> Out Bus Element8/1, Velocity Conversion/1
  Mach Number/1(Mach) -> Out Bus Element3/1
  Dynamic Pressure/1(qbar) -> Out Bus Element2/1
  Density Conversion/1 -> Dynamic Pressure/2(rho)
  In Bus Element3/1 -> Dynamic Pressure/1(Vt)  "Vt (ft/s)"
  In Bus Element4/1 -> Mach Number/1(Vt)  "Vt (ft/s)"
  Velocity Conversion/1 -> Mach Number/2(a)
  COESA Atmosphere Model/3 -> Pressure Altitude/1
  r2d1/1 -> Dryden Wind Turbulence Model (Continuous (+q +r))/1, Wind Shear Model/1  "h(ft)"
  In Bus Element2/1 -> r2d1/1
  In Bus Element5/1 -> Discrete Wind Gust Model/1, Dryden Wind Turbulence Model (Continuous (+q +r))/2  "Vt (ft/s)"
  In Bus Element/1 -> Wind Shear Model/2, Dryden Wind Turbulence Model (Continuous (+q +r))/3
  Dryden Wind Turbulence Model (Continuous (+q +r))/1 -> Sum/2
  Discrete Wind Gust Model/1 -> Sum/3
  Wind Shear Model/1 -> Sum/1
  Dryden Wind Turbulence Model (Continuous (+q +r))/2 -> Manual Switch1/1  "WindAngularRates"
  Sum/1 -> Manual Switch/2  "WindVelocity"
  Manual Switch/1 -> Out Bus Element9/1
  no wind/1 -> Manual Switch/1
  Manual Switch1/1 -> Out Bus Element10/1
  no wind1/1 -> Manual Switch1/2

== system Linearization/Rotation Speed(TVC OFF)OK ==
  pqr command : Inport
  In Bus Element : Inport  Port=2  PortName=PlantData  Element=Vt
  Constant : Constant  Value=0
  If : If  IfExpression=u1 > 220  ElseIfExpressions=220 >= u1 >= 135
  If Action Subsystem : Subsystem  TreatAsAtomicUnit=on
  If Action Subsystem1 : Subsystem  TreatAsAtomicUnit=on
  Merge : Merge
  Terminator1 : Terminator
  Output : Outport
  wires:
  If/1 -> If Action Subsystem/Action
  Constant/1 -> If Action Subsystem1/1(In1)
  If Action Subsystem1/1(Out1) -> Merge/2
  If Action Subsystem/1(Out1) -> Merge/1
  pqr command/1 -> If Action Subsystem/1(pqr command)
  Merge/1 -> Output/1
  In Bus Element/1 -> If/1
  If/2 -> If Action Subsystem1/Action
  If/3 -> Terminator1/1
